simulink model "Prototype2C"  (R2015a)
settings: Solver=ode45  StartTime=0.0  StopTime=10.0  RelTol=1e-3
undefined symbols (not defined in the file): gray, Rec, SDTV
libraries: visionanalysis x2, visiontransforms x2, visionconversions x1, visiontextngfix x1, visionstatistics x1, dspvision x1, visionsinks x1
settings Model: Creator=hoanga  LastModifiedBy=Andrew

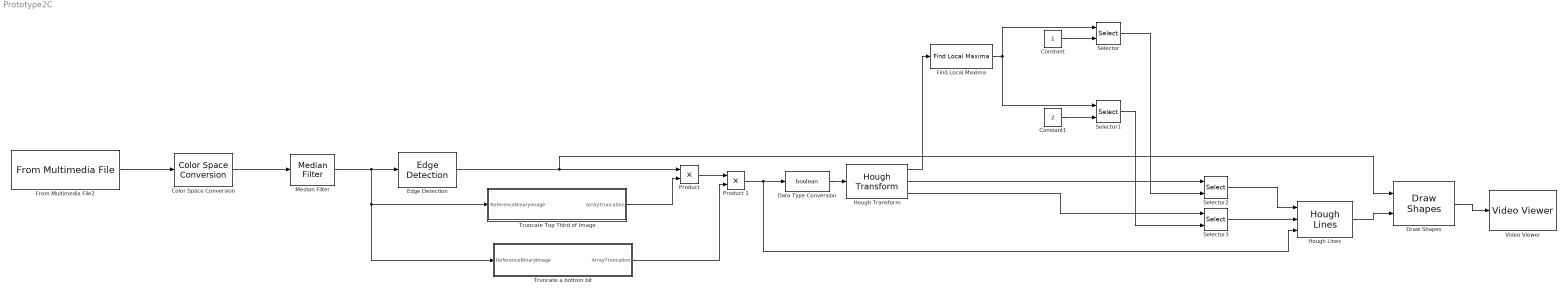
== system Prototype2C ==
  Color Space Conversion : visionconversions/Color Space  Conversion  conversion=Obsolete  conversionActive=R'G'B' to intensity  wp_str=D65  rec=Rec. 601 (SDTV)  sys=1125/60/2:1  imagePorts=One multidimensional signal
  Constant : Constant
  Constant1 : Constant  Value=2
  Data Type Conversion : DataTypeConversion  OutDataTypeStr=boolean
  Draw Shapes : visiontextngfix/Draw Shapes  shape=Lines  fill=on  lineWidth=4  fillClrSource=Specify via dialog  display=White  intensity=200  color=[255 0 0]  opacity=0.6  viewport=Entire image  antialiasing=off  inType=Obsolete  imagePorts=One multidimensional signal  prodOutputMode=Binary point scaling  prodOutputWordLength=32  prodOutputFracLength=14  memoryMode=Specify word length  memoryWordLength=16  memoryFracLength=14  roundingMode=Floor  overflowMode=off
  Edge Detection : visionanalysis/Edge Detection  method=Sobel  outputType=Binary image  userDefinedThreshold=off  thresholdSource=Input port  threshold=20  thresholdTuning=4  edgeThinning=off  threshold_canny=[0.25 0.60]  autoPercent=70  sigma=1  prodOutputMode=Binary point scaling  prodOutputWordLength=32  prodOutputFracLength=8  roundingMode=Floor  overflowMode=off
  Find Local Maxima : visionstatistics/Find Local Maxima  num_peaks=1  nhood_size=[5 7]  src_thresh=Obsolete9b  src_thresh_inuse=Specify via dialog  threshold=10  inputIsHough=on  dt_peak=uint32  isOutVarDim=on  dt_count=uint32
  From Multimedia File2 : dspvision/From Multimedia File  inputFilename=C:\Users\Andrew\Desktop\101MEDIA\PPG07820.MOV  loop=on  numPlays=inf  outputStreams=Video only  videoDataType=single  audioDataType=int16  inheritSampleTime=on  userDefinedSampleTime=1/30  noAudioOutput=off  isIntensityVideo=off  fourcc=RGB  colorVideoFormat=One multidimensional signal  outputEOF=off  dataOrg=Column-major  audioFrameSize=1024  computeAudioFrameSize=off  outSamplingMode=Sample based
  Hough Lines : visiontransforms/Hough Lines  sineCompMethod=Trigonometric function  thetaRes=pi/180  firstCoeffMode=Specify word length  firstCoeffWordLength=16  firstCoeffFracLength=15  prodOutputMode=Binary point scaling  prodOutputWordLength=32  prodOutputFracLength=16  roundingMode=Nearest  overflowMode=on
  Hough Transform : visiontransforms/Hough Transform  theta_res=pi/180  rho_res=1  out_theta_rho=on  outdtmode=double  firstCoeffMode=Binary point scaling  firstCoeffWordLength=16  firstCoeffFracLength=14  secondCoeffMode=Binary point scaling  secondCoeffWordLength=32  secondCoeffFracLength=16  outputMode=Binary point scaling  outputWordLength=16  outputFracLength=0  accumMode=Binary point scaling  accumWordLength=32  accumFracLength=20  prodOutputMode=Binary point scaling  prodOutputWordLength=32  prodOutputFracLength=20  memoryMode=Binary point scaling  memoryWordLength=32  memoryFracLength=16  roundingMode=Nearest  overflowMode=on
  Median Filter : visionanalysis/Median Filter  nghbood=[3 3]  outSize=Same as input port I  padType=Constant  padSrc=Specify via dialog  padVal=0  roundingMode=Floor  overflowMode=off
  "Product " : Product
  Product 1 : Product
  Selector : Selector  InputPortWidth=2  IndexOptions=Index vector (port)
  Selector1 : Selector  InputPortWidth=2  IndexOptions=Index vector (port)
  Selector2 : Selector  NumberOfDimensions=2  InputPortWidth=2  IndexOptions=Select all,Index vector (port)  Indices=1,1  OutputSizes=1,1
  Selector3 : Selector  NumberOfDimensions=2  InputPortWidth=2  IndexOptions=Select all,Index vector (port)  Indices=1,1  OutputSizes=1,1
  Truncate Top Third of Image : MATLAB Function  TreatAsAtomicUnit=on
  Truncate a bottom bit : MATLAB Function  TreatAsAtomicUnit=on
  Video Viewer : visionsinks/Video Viewer  inputType=Obsolete7b  imagePorts=One multidimensional signal  useColorMap=off  colormapValue=gray(256)  specRange=off  minInputVal=0  maxInputVal=255  FigPos=[1 1038 1920 939]  AxisZoom=on  trueSizedOnce=off  OpenAtMdlStart=on  DefaultConfigurationName=vipscopes.VideoViewerScopeCfg
  wires:
  Truncate Top Third of Image/1(ArrayTruncation) -> "Product "/2
  Edge Detection/1 -> Draw Shapes/1, "Product "/1
  "Product "/1 -> Product 1/1
  Truncate a bottom bit/1(ArrayTruncation) -> Product 1/2
  Draw Shapes/1 -> Video Viewer/1
  Hough Transform/1 -> Find Local Maxima/1
  Hough Lines/1 -> Draw Shapes/2
  Find Local Maxima/1 -> Selector/1, Selector1/1
  Constant/1 -> Selector/2
  Constant1/1 -> Selector1/2
  Selector/1 -> Selector2/2
  Selector1/1 -> Selector3/2
  Hough Transform/2 -> Selector2/1
  Hough Transform/3 -> Selector3/1
  Selector3/1 -> Hough Lines/2
  Selector2/1 -> Hough Lines/1
  Product 1/1 -> Data Type Conversion/1, Hough Lines/3
  Data Type Conversion/1 -> Hough Transform/1
  From Multimedia File2/1 -> Color Space Conversion/1
  Color Space Conversion/1 -> Median Filter/1
  Median Filter/1 -> Truncate a bottom bit/1(ReferenceBinaryImage), Truncate Top Third of Image/1(ReferenceBinaryImage), Edge Detection/1

== matlab function Prototype2C/Truncate a bottom bit ==
  data: ReferenceBinaryImage input; ArrayTruncation output
function ArrayTruncation = fcn(ReferenceBinaryImage)

%This function truncates the image you are processing by O variable fraction.
% In this case, O was set to 3 and deletes the first third of the flattened
% 2D array.

O = 9/10;

[x,y] = size(ReferenceBinaryImage);
matrix = ones(x, y);

for i = x*O:x
    for j = 1:y
        matrix(i,j) = 0;
    end
end

ArrayTruncation = matrix;

end

== matlab function Prototype2C/Truncate Top Third of Image ==
  data: ReferenceBinaryImage input; ArrayTruncation output
function ArrayTruncation = fcn(ReferenceBinaryImage)

%This function truncates the image you are processing by O variable fraction.
% In this case, O was set to 3 and deletes the first third of the flattened
% 2D array.

O = 4/10; %1/3 1/2 4/10

[x,y] = size(ReferenceBinaryImage);
matrix = zeros(x, y);

for i = x*O:x
    for j = 1:y
        matrix(i,j) = 1;
    end
end

ArrayTruncation = matrix;

end
